simulink model "model_PID_regulator"  (Simulink 7.1)
settings: Solver=ode45  StartTime=0.0  StopTime=20  RelTol=1e-3
settings Model: Creator=ahp  LastModifiedBy=ahp

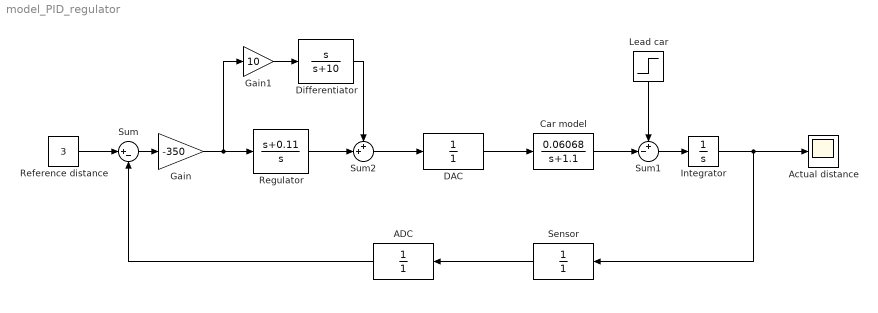
== system model_PID_regulator ==
  ADC : TransferFcn  Orientation=left  Denominator=[1]
  Actual distance : Scope
      settings: TimeRange=20  YMin=2  YMax=4
  Car model : TransferFcn  Numerator=[0.06068]  Denominator=[1 1.1]
  DAC : TransferFcn  Denominator=[1]
  Differentiator : TransferFcn  Numerator=[1 0]  Denominator=[1 10]
  Gain : Gain  Gain=-350  ParameterDataType=sfix(16)  ParameterScaling=2^0  OutDataType=sfix(16)  OutScaling=2^0
  Gain1 : Gain  Gain=10  ParameterDataType=sfix(16)  ParameterScaling=2^0  OutDataType=sfix(16)  OutScaling=2^0
  Integrator : Integrator
  Lead car : Step  Orientation=down  Time=0  SampleTime=0
  Reference distance : Constant  Value=3  OutDataType=sfix(16)  OutScaling=2^0
  Regulator : TransferFcn  Numerator=[1 0.11]  Denominator=[1 0]
  Sensor : TransferFcn  Orientation=left  Denominator=[1]
  Sum : Sum  Inputs=|+-  OutDataType=sfix(16)  OutScaling=2^0
  Sum1 : Sum  Inputs=+-|  OutDataType=sfix(16)  OutScaling=2^0
  Sum2 : Sum  Inputs=++|  OutDataType=sfix(16)  OutScaling=2^0
  wires:
  Reference distance/1 -> Sum/1
  Car model/1 -> Sum1/2
  Lead car/1 -> Sum1/1
  Sum1/1 -> Integrator/1
  Integrator/1 -> Actual distance/1, Sensor/1
  ADC/1 -> Sum/2
  DAC/1 -> Car model/1
  Sensor/1 -> ADC/1
  Sum2/1 -> DAC/1
  Sum/1 -> Gain/1
  Gain/1 -> Regulator/1, Gain1/1
  Regulator/1 -> Sum2/2
  Differentiator/1 -> Sum2/1
  Gain1/1 -> Differentiator/1
